simulink model "comprehensive_model_with_rocks_trial"  (R2019a)
settings: Solver=FixedStepAuto  StartTime=0.0  StopTime=15  FixedStep=0.001  RelTol=1e-3
PreLoadFcn:
  | load('tumbleweed_constants.mat')
values from neighbouring files (symbols this model uses):
  Ar = 0.785398163397    [tumbleweed_constants.mat]
  CD = 0.8    [tumbleweed_constants.mat]
  d = 0.65    [tumbleweed_constants.mat]
  g = 9.81    [tumbleweed_constants.mat]
  Ixx = 1.29    [tumbleweed_constants.mat]
  Iyy = 1.29    [tumbleweed_constants.mat]
  Izz = 1.29    [tumbleweed_constants.mat]
  m = 1    [tumbleweed_constants.mat]
  maxr = 0.45    [tumbleweed_constants.mat]
  mf = 14    [tumbleweed_constants.mat]
  minr = 0.2    [tumbleweed_constants.mat]
  mu0 = 0.02    [tumbleweed_constants.mat]
  muk = 0.5    [tumbleweed_constants.mat]
  must = 0.8    [tumbleweed_constants.mat]
  R = cylR*ones(size(Theta,1),size(Theta,2))    [d3_animate.m]    (also in tumbleweed_constants.mat = 0.5)
  rest_coeff = 0.6    [tumbleweed_constants.mat]
  rho = 1.2    [tumbleweed_constants.mat]
  ts = 0.5    [tumbleweed_constants.mat]
  v_thres = 0.0001    [tumbleweed_constants.mat]
  vmax = 0.2    [tumbleweed_constants.mat]
  YY = 50    [tumbleweed_constants.mat]
libraries: simulink x2
(part 4 of 9)

== matlab function comprehensive_model_with_rocks_trial/bouncing_model/onsurface_model/MATLAB Function5 ==
  data: t input; jAp input; states_from_memory input; states_internal input; r_AO0 input; roll_reset_flag input; surf_num_memory input; surf_num_internal input; rock_cents input; rock_radi input; switch_t input; OwT_OvAO0 output; R parameter; r_AO0 output; q output; roll_reset_flag output; reset_states output; reset_states input; surf_num output
function  [OwT_OvAO0, r_AO0, q,roll_reset_flag,reset_states,surf_num] = init_cond_supp(t,jAp, states_from_memory, states_internal,r_AO0, roll_reset_flag,surf_num_memory,surf_num_internal,rock_cents,rock_radi,switch_t, R, reset_states)
if t == 115.737
    disp(t)
end
if (t - switch_t) == 0
    roll_reset_flag = 1;
    states0 = states_from_memory;
    surf_num = surf_num_memory;
else
    states0 = states_internal;
    if mod(t,0.001) == 0
        surf_num = surf_num_internal;
    else
        surf_num = surf_num_memory;
    end
end
    
O_w_T = states0(1:3,1);
O_v_TO = states0(4:6,1);
r_TO = states0(7:9,1);
q = states0(10:13,1);
rock_radi = rock_radi.';


kO = [0;0;1];
jO = [0;1;0];
iO = [1;0;0];
point_on_surf =  zeros(2,1);
smallest_dist = 0;
if (roll_reset_flag == 1 && surf_num == 0)
    [point_on_surf, smallest_dist] = dist_calc(r_TO);
%     point_on_surf = [r_TO(1);r_TO(2)];
%     smallest_dist = r_TO(3);
    z_c = surf_eq(point_on_surf(1),point_on_surf(2),r_TO);
    r_AO0 = [point_on_surf;z_c];
elseif (roll_reset_flag == 1 && surf_num > 0)
    kR = (r_TO - rock_cents(:,surf_num))/norm(r_TO -  rock_cents(:,surf_num));
    point_on_rock = rock_cents(:,surf_num) + rock_radi(1,surf_num)*kR;
    r_AO0 = point_on_rock;
end

if surf_num == 0
    par_diffs = par_diffs_calc(r_AO0);
else
    par_diffs = rock_pardiffs_calc(r_AO0, rock_cents(:,surf_num)');
end

vx = O_v_TO(1); vy = O_v_TO(2); vz = O_v_TO(3);
fx = par_diffs(1);
fy = par_diffs(2);
fz = par_diffs(3);
fxx = par_diffs(4);
fxy = par_diffs(5);
fxz = par_diffs(6);
fyy = par_diffs(7);
fyz = par_diffs(8);
fzz = par_diffs(9);
fxxx = par_diffs(10);
fxxy = par_diffs(11);
fxxz = par_diffs(12);
fxyy = par_diffs(13);
fxyz = par_diffs(14);
fxzz = par_diffs(15);
fyyy = par_diffs(16);
fyyz = par_diffs(17);
fyzz = par_diffs(18);
fzzz = par_diffs(19);




q0 = q(1); q1 = q(2); q2 = q(3); q3 = q(4);


T_c_O = [q0^2 + q1^2 - q2^2 - q3^2, 2*(q1*q2 + q0*q3), 2*(q1*q3 - q0*q2);...
       2*(q1*q2 - q0*q3), q0^2 - q1^2 + q2^2 - q3^2, 2*(q2*q3 + q0*q1);...
       2*(q1*q3 + q0*q2), 2*(q2*q3 - q0*q1), q0^2 - q1^2 - q2^2 + q3^2];

c11 = T_c_O(1,1);c12 = T_c_O(1,2); c13 = T_c_O(1,3);
c21 = T_c_O(2,1);c22 = T_c_O(2,2); c23 = T_c_O(2,3);
c31 = T_c_O(3,1);c32 = T_c_O(3,2); c33 = T_c_O(3,3);




%z - cos(x/4)-1 = 0;
%- x^2 - y^2 = 0;

if(abs(fx)<=1e-20 && abs(fy) <= 1e-20)
    kA = kO;
    O_c_A = eye(3);
    A_c_O = eye(3);
    flag = 1;
else
    kA = [fx;fy;fz]/norm([fx;fy;fz]);
    jA = cross(kO,kA)/norm(cross(kO,kA));
    flag = 1;
    if((jAp.')*(jA) < 0)
        jA = -jA;
        flag = 2;
    end
    iA = cross(jA,kA);
    A_c_O = [iA'*iO, iA'*jO, iA'*kO; jA'*iO, jA'*jO, jA'*kO; kA'*iO, kA'*jO, kA'*kO];
    O_c_A = transpose(A_c_O);
end


if flag == 1
    
% OvAO_coeffs = ...
% [fx, fy, fz;...
% ((fx*fz*(fx^2 + fy^2 + fz^2)^(3/2) - R*fxz*(fx^2 + fy^2)^2 + R*fx*fxx*fz^3 + R*fxy*fy*fz^3 - R*fxz*fz^2*(fx^2 + fy^2) + R*fx*fxx*fz*(fx^2 + fy^2) + R*fxy*fy*fz*(fx^2 + fy^2))/((fx^2 + fy^2)^(1/2)*(fx^2 + fy^2 + fz^2)^2)),            ((fy*fz*(fx^2 + fy^2 + fz^2)^(3/2) - R*fyz*(fx^2 + fy^2)^2 + R*fx*fxy*fz^3 + R*fy*fyy*fz^3 - R*fyz*fz^2*(fx^2 + fy^2) + R*fx*fxy*fz*(fx^2 + fy^2) + R*fy*fyy*fz*(fx^2 + fy^2))/((fx^2 + fy^2)^(1/2)*(fx^2 + fy^2 + fz^2)^2)),               ((R*fx*fxz*fz^3 - R*fzz*(fx^2 + fy^2)^2 - (fx^2 + fy^2)*(fx^2 + fy^2 + fz^2)^(3/2) + R*fy*fyz*fz^3 - R*fz^2*fzz*(fx^2 + fy^2) + R*fx*fxz*fz*(fx^2 + fy^2) + R*fy*fyz*fz*(fx^2 + fy^2))/((fx^2 + fy^2)^(1/2)*(fx^2 + fy^2 + fz^2)^2));...
% (-(fy*(fx^2 + fy^2 + fz^2)^(1/2) - R*fx*fxy + R*fxx*fy)/((fx^2 + fy^2)^(1/2)*(fx^2 + fy^2 + fz^2)^(1/2))),                                                                                                                               ((fx*(fx^2 + fy^2 + fz^2)^(1/2) + R*fx*fyy - R*fxy*fy)/((fx^2 + fy^2)^(1/2)*(fx^2 + fy^2 + fz^2)^(1/2))),                                                                                                                                   ((R*fx*fyz - R*fxz*fy)/((fx^2 + fy^2)^(1/2)*(fx^2 + fy^2 + fz^2)^(1/2)))];
% 
% OvAO_consts = ...
% [0;...
% - (fx*fz*vx*(fx^2 + fy^2 + fz^2)^(3/2) - vz*(fx^2 + fy^2)*(fx^2 + fy^2 + fz^2)^(3/2) + fy*fz*vy*(fx^2 + fy^2 + fz^2)^(3/2))/((fx^2 + fy^2)^(1/2)*(fx^2 + fy^2 + fz^2)^2);...
% - (fx*vy*(fx^2 + fy^2 + fz^2)^(1/2) - fy*vx*(fx^2 + fy^2 + fz^2)^(1/2))/((fx^2 + fy^2)^(1/2)*(fx^2 + fy^2 + fz^2)^(1/2))];
%   

OvAO_coeffs = ...
 [(((fx^2 + fy^2 + fz^2)^(3/2) + R*fxx*fy^2 + R*fxx*fz^2 - R*fx*fxy*fy - R*fx*fxz*fz)/(fx^2 + fy^2 + fz^2)^(3/2)),       ((R*fxy*fy^2 - R*fx*fyy*fy + R*fxy*fz^2 - R*fx*fyz*fz)/(fx^2 + fy^2 + fz^2)^(3/2)),                                     ((R*fxz*fy^2 - R*fx*fyz*fy + R*fxz*fz^2 - R*fx*fzz*fz)/(fx^2 + fy^2 + fz^2)^(3/2));...
 ((R*fxy*fx^2 - R*fxx*fy*fx + R*fxy*fz^2 - R*fxz*fy*fz)/(fx^2 + fy^2 + fz^2)^(3/2)),                                     (((fx^2 + fy^2 + fz^2)^(3/2) + R*fx^2*fyy + R*fyy*fz^2 - R*fx*fxy*fy - R*fy*fyz*fz)/(fx^2 + fy^2 + fz^2)^(3/2)),        ((R*fyz*fx^2 - R*fxz*fy*fx + R*fyz*fz^2 - R*fy*fzz*fz)/(fx^2 + fy^2 + fz^2)^(3/2));...
 ((R*fxz*fx^2 - R*fxx*fz*fx + R*fxz*fy^2 - R*fxy*fz*fy)/(fx^2 + fy^2 + fz^2)^(3/2)),                                     ((R*fyz*fx^2 - R*fxy*fz*fx + R*fyz*fy^2 - R*fyy*fz*fy)/(fx^2 + fy^2 + fz^2)^(3/2)),                                     (((fx^2 + fy^2 + fz^2)^(3/2) + R*fx^2*fzz + R*fy^2*fzz - R*fx*fxz*fz - R*fy*fyz*fz)/(fx^2 + fy^2 + fz^2)^(3/2))];

OvAO_consts = ...
  [-vx;...
   -vy;...
   -vz];


else
    
% OvAO_coeffs = ...  
% [fx, fy, fz;...
% (-(fx*fz*(fx^2 + fy^2 + fz^2)^(3/2) - R*fxz*(fx^2 + fy^2)^2 + R*fx*fxx*fz^3 + R*fxy*fy*fz^3 - R*fxz*fz^2*(fx^2 + fy^2) + R*fx*fxx*fz*(fx^2 + fy^2) + R*fxy*fy*fz*(fx^2 + fy^2))/((fx^2 + fy^2)^(1/2)*(fx^2 + fy^2 + fz^2)^2)),           (-(fy*fz*(fx^2 + fy^2 + fz^2)^(3/2) - R*fyz*(fx^2 + fy^2)^2 + R*fx*fxy*fz^3 + R*fy*fyy*fz^3 - R*fyz*fz^2*(fx^2 + fy^2) + R*fx*fxy*fz*(fx^2 + fy^2) + R*fy*fyy*fz*(fx^2 + fy^2))/((fx^2 + fy^2)^(1/2)*(fx^2 + fy^2 + fz^2)^2)),              (-(R*fx*fxz*fz^3 - R*fzz*(fx^2 + fy^2)^2 - (fx^2 + fy^2)*(fx^2 + fy^2 + fz^2)^(3/2) + R*fy*fyz*fz^3 - R*fz^2*fzz*(fx^2 + fy^2) + R*fx*fxz*fz*(fx^2 + fy^2) + R*fy*fyz*fz*(fx^2 + fy^2))/((fx^2 + fy^2)^(1/2)*(fx^2 + fy^2 + fz^2)^2));...
% ((fy*(fx^2 + fy^2 + fz^2)^(1/2) - R*fx*fxy + R*fxx*fy)/((fx^2 + fy^2)^(1/2)*(fx^2 + fy^2 + fz^2)^(1/2))),                                                                                                                                (-(fx*(fx^2 + fy^2 + fz^2)^(1/2) + R*fx*fyy - R*fxy*fy)/((fx^2 + fy^2)^(1/2)*(fx^2 + fy^2 + fz^2)^(1/2))),                                                                                                                                  (-(R*fx*fyz - R*fxz*fy)/((fx^2 + fy^2)^(1/2)*(fx^2 + fy^2 + fz^2)^(1/2)))];      
%  
% OvAO_consts = ...
% [0;...
% (fx*fz*vx*(fx^2 + fy^2 + fz^2)^(3/2) - vz*(fx^2 + fy^2)*(fx^2 + fy^2 + fz^2)^(3/2) + fy*fz*vy*(fx^2 + fy^2 + fz^2)^(3/2))/((fx^2 + fy^2)^(1/2)*(fx^2 + fy^2 + fz^2)^2);...
% (fx*vy*(fx^2 + fy^2 + fz^2)^(1/2) - fy*vx*(fx^2 + fy^2 + fz^2)^(1/2))/((fx^2 + fy^2)^(1/2)*(fx^2 + fy^2 + fz^2)^(1/2))];

OvAO_coeffs = ...
   [(((fx^2 + fy^2 + fz^2)^(3/2) + R*fxx*fy^2 + R*fxx*fz^2 - R*fx*fxy*fy - R*fx*fxz*fz)/(fx^2 + fy^2 + fz^2)^(3/2)),              ((R*fxy*fy^2 - R*fx*fyy*fy + R*fxy*fz^2 - R*fx*fyz*fz)/(fx^2 + fy^2 + fz^2)^(3/2)),                                     ((R*fxz*fy^2 - R*fx*fyz*fy + R*fxz*fz^2 - R*fx*fzz*fz)/(fx^2 + fy^2 + fz^2)^(3/2));...
    ((R*fxy*fx^2 - R*fxx*fy*fx + R*fxy*fz^2 - R*fxz*fy*fz)/(fx^2 + fy^2 + fz^2)^(3/2)),                                           (((fx^2 + fy^2 + fz^2)^(3/2) + R*fx^2*fyy + R*fyy*fz^2 - R*fx*fxy*fy - R*fy*fyz*fz)/(fx^2 + fy^2 + fz^2)^(3/2)),        ((R*fyz*fx^2 - R*fxz*fy*fx + R*fyz*fz^2 - R*fy*fzz*fz)/(fx^2 + fy^2 + fz^2)^(3/2));...
    ((R*fxz*fx^2 - R*fxx*fz*fx + R*fxz*fy^2 - R*fxy*fz*fy)/(fx^2 + fy^2 + fz^2)^(3/2)),                                           ((R*fyz*fx^2 - R*fxy*fz*fx + R*fyz*fy^2 - R*fyy*fz*fy)/(fx^2 + fy^2 + fz^2)^(3/2)),                                     (((fx^2 + fy^2 + fz^2)^(3/2) + R*fx^2*fzz + R*fy^2*fzz - R*fx*fxz*fz - R*fy*fyz*fz)/(fx^2 + fy^2 + fz^2)^(3/2))];

OvAO_consts = ...
  [-vx;...
   -vy;...
   -vz];

end

if (abs(fx) <= 1e-20 && abs(fy) <= 1e-20 )
    O_v_AO = O_v_TO;
else
O_v_AO = -inv(OvAO_coeffs)*OvAO_consts;
end
O_v_AOa = A_c_O*O_v_AO;
if O_v_AOa(3) <= 0.008 && O_v_AOa(3) >= -0.008
    O_v_AOa(3) = 0;
    O_v_AO = O_c_A*O_v_AOa;
end
% if norm([O_v_AO(1);O_v_AO(2)]) < 0.00 
%     O_v_AO(1) = 0;
%     O_v_AO(2) = 0;
% end
OwT_OvAO0 = [O_w_T;O_v_AO];
if roll_reset_flag == 1
 reset_states = [O_w_T;O_v_AO;r_AO0;q];
end

end




function rock_pardiffs = rock_pardiffs_calc(point_on_rock, rock_center)
r_RO = point_on_rock; x_c = r_RO(1); y_c = r_RO(2); z_c = r_RO(3);
r_CO = rock_center';
fx = 2*(x_c - r_CO(1));
fy = 2*(y_c - r_CO(2));
fz = 2*(z_c - r_CO(3));
fxx = 2;
fxy = 0;
fxz = 0;
fyy = 2;
fyz = 0;
fzz = 2;
fxxx = 0;
fxxy = 0;
fxxz = 0;
fxyy = 0;
fxyz = 0;
fxzz = 0;
fyyy = 0;
fyyz = 0;
fyzz = 0;
fzzz = 0;
rock_pardiffs = [fx;fy;fz;fxx;fxy;fxz;fyy;fyz;fzz;fxxx;fxxy;fxxz;fxyy;fxyz;fxzz;fyyy;fyyz;fyzz;fzzz];
end



function par_diffs = par_diffs_calc(r_AO)

x_c = r_AO(1);
y_c = r_AO(2);
z_c = r_AO(3);

fx = 0;%4*exp(- (x_c - 5)^2/36 - y_c^2/36)*(x_c/18 - 5/18) - 6*exp(- (x_c - 5)^2/16 - y_c^2/16)*(x_c/8 - 5/8);
fy = 0;%(2*y_c*exp(- (x_c - 5)^2/36 - y_c^2/36))/9 - (3*y_c*exp(- (x_c - 5)^2/16 - y_c^2/16))/4;
fz = 1;
fxx = 0;%(2*exp(- (x_c - 5)^2/36 - y_c^2/36))/9 - (3*exp(- (x_c - 5)^2/16 - y_c^2/16))/4 + 6*exp(- (x_c - 5)^2/16 - y_c^2/16)*(x_c/8 - 5/8)^2 - 4*exp(- (x_c - 5)^2/36 - y_c^2/36)*(x_c/18 - 5/18)^2;
fxy = 0;%(3*y_c*exp(- (x_c - 5)^2/16 - y_c^2/16)*(x_c/8 - 5/8))/4 - (2*y_c*exp(- (x_c - 5)^2/36 - y_c^2/36)*(x_c/18 - 5/18))/9;
fxz = 0;
fyy = 0;%(2*exp(- (x_c - 5)^2/36 - y_c^2/36))/9 - (3*exp(- (x_c - 5)^2/16 - y_c^2/16))/4 + (3*y_c^2*exp(- (x_c - 5)^2/16 - y_c^2/16))/32 - (y_c^2*exp(- (x_c - 5)^2/36 - y_c^2/36))/81;
fyz = 0;
fzz = 0;
fxxx = 0;%(3*exp(- (x_c - 5)^2/16 - y_c^2/16)*(x_c/8 - 5/8))/4 + 6*exp(- (x_c - 5)^2/16 - y_c^2/16)*(x_c/32 - 5/32) - (2*exp(- (x_c - 5)^2/36 - y_c^2/36)*(x_c/18 - 5/18))/9 - 4*exp(- (x_c - 5)^2/36 - y_c^2/36)*(x_c/162 - 5/162) - 6*exp(- (x_c - 5)^2/16 - y_c^2/16)*(x_c/8 - 5/8)^3 + 4*exp(- (x_c - 5)^2/36 - y_c^2/36)*(x_c/18 - 5/18)^3;
fxxy = 0;%(3*y_c*exp(- (x_c - 5)^2/16 - y_c^2/16))/32 - (y_c*exp(- (x_c - 5)^2/36 - y_c^2/36))/81 - (3*y_c*exp(- (x_c - 5)^2/16 - y_c^2/16)*(x_c/8 - 5/8)^2)/4 + (2*y_c*exp(- (x_c - 5)^2/36 - y_c^2/36)*(x_c/18 - 5/18)^2)/9;
fxxz = 0;
fxyy = 0;%(3*exp(- (x_c - 5)^2/16 - y_c^2/16)*(x_c/8 - 5/8))/4 - (2*exp(- (x_c - 5)^2/36 - y_c^2/36)*(x_c/18 - 5/18))/9 - (3*y_c^2*exp(- (x_c - 5)^2/16 - y_c^2/16)*(x_c/8 - 5/8))/32 + (y_c^2*exp(- (x_c - 5)^2/36 - y_c^2/36)*(x_c/18 - 5/18))/81;
fxyz = 0;
fxzz = 0;
fyyy = 0;%(9*y_c*exp(- (x_c - 5)^2/16 - y_c^2/16))/32 - (y_c*exp(- (x_c - 5)^2/36 - y_c^2/36))/27 - (3*y_c^3*exp(- (x_c - 5)^2/16 - y_c^2/16))/256 + (y_c^3*exp(- (x_c - 5)^2/36 - y_c^2/36))/1458;
fyyz = 0;
fyzz = 0;
fzzz = 0;

% fx = -x_c;
% fy = 1;
% fz = z_c;
% fxx = -1;
% fxy = 0;
% fxz = 0;
% fyy = 0;
% fyz = 0;
% fzz = 1;
% fxxx = 0;
% fxxy = 0;
% fxxz = 0;
% fxyy = 0;
% fxyz = 0;
% fxzz = 0;
% fyyy = 0;
% fyyz = 0;
% fyzz = 0;
% fzzz = 0;

par_diffs = [fx;fy;fz;fxx;fxy;fxz;fyy;fyz;fzz;fxxx;fxxy;fxxz;fxyy;fxyz;fxzz;fyyy;fyyz;fyzz;fzzz];
end

function z_c = surf_eq(x_c, y_c, r_TO)
% if r_TO(3) >= 0
%     if x_c^2 - 2*y_c < 0
%         z_c = 0;
%     else
%     z_c = sqrt(x_c^2 - 2*y_c);
%     end
% else
%     if x_c^2 - 2*y_c < 0
%         z_c = 0;
%     else
%     z_c = -sqrt(x_c^2 - 2*y_c);
%     end
% end
z_c = 0;%(4*exp(-((x_c-5)^2 + (y_c)^2)/(6^2))-6*exp(-((x_c-5)^2 + (y_c)^2)/(4^2)));%(-1*exp(-((x_c - 10)^2 + (y_c - 10)^2)/2^2) -5*exp(-((x_c - 10)^2 + (y_c - 15)^2)/5^2) + 5*exp(-((x_c - 10)^2 + (y_c + 10)^2)/5^2) - 3*exp(-((x_c - 20)^2 + (y_c +5)^2)/4^2) - 5*exp(-((x_c - 40)^2 + (y_c -10)^2)/6^2));
end

== matlab function comprehensive_model_with_rocks_trial/bouncing_model/onsurface_model/MATLAB Function6 ==
  data: t input; switch_t input; states0 output; states input; states_from_memory input; point_on_rock output; rock_cents input; rock_radi input; rock_pardiffs output; rock_coll_flag output; R parameter; jAp input; surf_num input; surf_num output; roll_reset_flag input; reset_states input
function [states0, point_on_rock, rock_pardiffs, rock_coll_flag, surf_num] = collision_check(t, switch_t, states, states_from_memory,rock_cents, rock_radi,R, jAp, surf_num,roll_reset_flag,reset_states)
if t >= 88.46
    disp(t)
end
if (t - switch_t) == 0
    states0 = states_from_memory;
    O_w_T = states0(1:3,1);
    O_v_TO = states0(4:6,1);
    q = states0(10:13,1);
    r_TO = states0(7:9,1);
else
  states0 = states;
    if roll_reset_flag == 1
        states0 = reset_states;
    end
    O_w_T = states0(1:3,1);
    O_v_AO = states0(4:6,1);
    q = states0(10:13,1);
    r_AO = states0(7:9,1);
    [r_TO,  O_v_TO] = calc_OvTO_rTO(r_AO, O_v_AO, surf_num,rock_cents, jAp, R);
 end



rock_radi = rock_radi';
rock_coll_flag = 0;
rock_ind = 0;
kO = [0;0;1];
jO = [0;1;0];
iO = [1;0;0];

for i = 1:size(rock_cents,2)
    if i ~= surf_num
    if norm(r_TO - rock_cents(:,i)) <= rock_radi(1,i) + R + 0.001
        kR = (r_TO - rock_cents(:,i))/norm(r_TO -  rock_cents(:,i));   
       if(abs(kR(1))<=1e-10 && abs(kR(2))<=1e-10)
            kR = kO;
            jR = jO;
            iR = iO;
            O_c_R = eye(3);
            R_c_O = eye(3);
            flag = 1;
       else
        jR = cross(kO,kR)/norm(cross(kO,kR));
        flag = 1;
        if((jAp.')*(jR) < 0)
            jR = -jR;
            flag = 2;
        end
        iR = cross(jR,kR);
        R_c_O = [iR'*iO, iR'*jO, iR'*kO; jR'*iO, jR'*jO, jR'*kO; kR'*iO, kR'*jO, kR'*kO];
        O_c_R = transpose(R_c_O);
        end
    O_v_TOr = R_c_O*O_v_TO;  
        if O_v_TOr(3)< -0.001
                rock_coll_flag = 1;
                rock_ind = i;
        end
    end
    end
end

point_on_surf = [0;0];z_c = 0;
 smallest_dist = 0;
if surf_num ~= 0
     [point_on_surf, smallest_dist] = dist_calc(r_TO);
%     point_on_surf = [r_TO(1);r_TO(2)];
%     smallest_dist = r_TO(3);
    z_c = surf_eq(point_on_surf(1),point_on_surf(2),r_TO);
    if norm(r_TO - [point_on_surf;z_c]) <= R + 0.001  
                rock_coll_flag = 1;
                rock_ind = 0;
    end
end

if rock_coll_flag == 1
    if rock_ind == 0
        point_on_rock  = [point_on_surf;z_c];
        rock_pardiffs = surf_pardiffs_calc(point_on_rock);
%         fx = rock_pardiffs(1);
%         fy = rock_pardiffs(2);
%         fz = rock_pardiffs(3);
%         if(abs(fx)<=1e-20 && abs(fy) <= 1e-20)
%             kR = kO;
%             jR = jO;
%             iR = iO;
%             O_c_R = eye(3);
%             R_c_O = eye(3);
%         else
%             kR = [fx;fy;fz]/norm([fx;fy;fz]);
%             jR = cross(kO,kR)/norm(cross(kO,kR));
%         if((jRp.')*(jR) < 0)
%             jR = -jR;
%         end
%         iR = cross(jR,kR);
%         R_c_O = [iR'*iO, iR'*jO, iR'*kO; jR'*iO, jR'*jO, jR'*kO; kR'*iO, kR'*jO, kR'*kO];
%         O_c_R = transpose(R_c_O);
%         end
%         O_v_TOr = R_c_O*O_v_TO;  
%         if abs(O_v_TOr(3))<=0.001 && mod(t,0.001) == 0
%             surf_num = 0;
%         end
    if mod(t,0.001) == 0
        surf_num = 0;
    end
    else
        kR = (r_TO - rock_cents(:,rock_ind))/norm(r_TO -  rock_cents(:,rock_ind));
        point_on_rock = rock_cents(:,rock_ind) + rock_radi(1,rock_ind)*kR;
        rock_pardiffs = rock_pardiffs_calc(point_on_rock, rock_cents(:,rock_ind));
    end
else
    point_on_rock = [0;0;0];
    rock_pardiffs = zeros(19,1);
end


states0 = [O_w_T; O_v_TO; r_TO; q];
end









function [r_TO,  O_v_TO] = calc_OvTO_rTO(r_AO, O_v_AO, surf_num,rock_cents, jAp, R)
%change this everytime u change the function

x_dot = O_v_AO(1);
y_dot = O_v_AO(2);
z_dot = O_v_AO(3);

kO = [0;0;1];
jO = [0;1;0];
iO = [1;0;0];

%z - cos(x/4)-1 = 0;
%- x^2 - y^2 = 0;


if surf_num == 0
    par_diffs = surf_pardiffs_calc(r_AO);
else
    rock_center = rock_cents(:,surf_num);
    par_diffs = rock_pardiffs_calc(r_AO, rock_center);
end
fx = par_diffs(1);
fy = par_diffs(2);
fz = par_diffs(3);
fxx = par_diffs(4);
fxy = par_diffs(5);
fxz = par_diffs(6);
fyy = par_diffs(7);
fyz = par_diffs(8);
fzz = par_diffs(9);
fxxx = par_diffs(10);
fxxy = par_diffs(11);
fxxz = par_diffs(12);
fxyy = par_diffs(13);
fxyz = par_diffs(14);
fxzz = par_diffs(15);
fyyy = par_diffs(16);
fyyz = par_diffs(17);
fyzz = par_diffs(18);
fzzz = par_diffs(19);


if(abs(fx)<=1e-20 && abs(fy) <= 1e-20)
    kA = kO;
    jA = jO;
    O_c_A = eye(3);
    A_c_O = eye(3);
    flag = 1;
else
    kA = [fx;fy;fz]/norm([fx;fy;fz]);
    jA = cross(kO,kA)/norm(cross(kO,kA));
    flag = 1;
    if((jAp.')*(jA) < 0)
        jA = -jA;
        flag = 2;
    end
    iA = cross(jA,kA);
    A_c_O = [iA'*iO, iA'*jO, iA'*kO; jA'*iO, jA'*jO, jA'*kO; kA'*iO, kA'*jO, kA'*kO];
    O_c_A = transpose(A_c_O);
end
if flag == 1
    O_w_A = ...
    [-(fx*fxy*x_dot - fy*fxx*x_dot + fx*fyy*y_dot - fy*fxy*y_dot + fx*fyz*z_dot - fy*fxz*z_dot)/((fx^2 + fy^2)^(1/2)*(fx^2 + fy^2 + fz^2)^(1/2));...
     -(fx^2*fxz*x_dot + fy^2*fxz*x_dot + fx^2*fyz*y_dot + fy^2*fyz*y_dot + fx^2*fzz*z_dot + fy^2*fzz*z_dot - fx*fxx*fz*x_dot - fy*fz*fxy*x_dot - fx*fz*fxy*y_dot - fy*fz*fyy*y_dot - fx*fz*fxz*z_dot - fy*fz*fyz*z_dot)/((fx^2 + fy^2)^(1/2)*(fx^2 + fy^2 + fz^2));...
     (fz*(fx*fxy*x_dot - fy*fxx*x_dot + fx*fyy*y_dot - fy*fxy*y_dot + fx*fyz*z_dot - fy*fxz*z_dot))/((fx^2 + fy^2)*(fx^2 + fy^2 + fz^2)^(1/2))];
else
    O_w_A = ...
    [(fx*fxy*x_dot - fy*fxx*x_dot + fx*fyy*y_dot - fy*fxy*y_dot + fx*fyz*z_dot - fy*fxz*z_dot)/((fx^2 + fy^2)^(1/2)*(fx^2 + fy^2 + fz^2)^(1/2));...
     (fx^2*fxz*x_dot + fy^2*fxz*x_dot + fx^2*fyz*y_dot + fy^2*fyz*y_dot + fx^2*fzz*z_dot + fy^2*fzz*z_dot - fx*fxx*fz*x_dot - fy*fz*fxy*x_dot - fx*fz*fxy*y_dot - fy*fz*fyy*y_dot - fx*fz*fxz*z_dot - fy*fz*fyz*z_dot)/((fx^2 + fy^2)^(1/2)*(fx^2 + fy^2 + fz^2));...
     (fz*(fx*fxy*x_dot - fy*fxx*x_dot + fx*fyy*y_dot - fy*fxy*y_dot + fx*fyz*z_dot - fy*fxz*z_dot))/((fx^2 + fy^2)*(fx^2 + fy^2 + fz^2)^(1/2))];
end
if (abs(fx) <= 1e-20 && abs(fy) <= 1e-20)
    O_w_A = [0;0;0];
end
r_TO = r_AO + R*kA;

r_TA = [0;0;R];
O_v_TO = O_v_AO + O_c_A*cross(O_w_A, r_TA);
end










function rock_pardiffs = rock_pardiffs_calc(point_on_rock, rock_center)
r_RO = point_on_rock; x_c = r_RO(1); y_c = r_RO(2); z_c = r_RO(3);
r_CO = rock_center';
fx = 2*(x_c - r_CO(1));
fy = 2*(y_c - r_CO(2));
fz = 2*(z_c - r_CO(3));
fxx = 2;
fxy = 0;
fxz = 0;
fyy = 2;
fyz = 0;
fzz = 2;
fxxx = 0;
fxxy = 0;
fxxz = 0;
fxyy = 0;
fxyz = 0;
fxzz = 0;
fyyy = 0;
fyyz = 0;
fyzz = 0;
fzzz = 0;
rock_pardiffs = [fx;fy;fz;fxx;fxy;fxz;fyy;fyz;fzz;fxxx;fxxy;fxxz;fxyy;fxyz;fxzz;fyyy;fyyz;fyzz;fzzz];
end











function par_diffs = surf_pardiffs_calc(r_AO)
x_c = r_AO(1);
y_c = r_AO(2);
z_c = r_AO(3);

fx = 0;%4*exp(- (x_c - 5)^2/36 - y_c^2/36)*(x_c/18 - 5/18) - 6*exp(- (x_c - 5)^2/16 - y_c^2/16)*(x_c/8 - 5/8);
fy = 0;%(2*y_c*exp(- (x_c - 5)^2/36 - y_c^2/36))/9 - (3*y_c*exp(- (x_c - 5)^2/16 - y_c^2/16))/4;
fz = 1;
fxx = 0;%(2*exp(- (x_c - 5)^2/36 - y_c^2/36))/9 - (3*exp(- (x_c - 5)^2/16 - y_c^2/16))/4 + 6*exp(- (x_c - 5)^2/16 - y_c^2/16)*(x_c/8 - 5/8)^2 - 4*exp(- (x_c - 5)^2/36 - y_c^2/36)*(x_c/18 - 5/18)^2;
fxy = 0;%(3*y_c*exp(- (x_c - 5)^2/16 - y_c^2/16)*(x_c/8 - 5/8))/4 - (2*y_c*exp(- (x_c - 5)^2/36 - y_c^2/36)*(x_c/18 - 5/18))/9;
fxz = 0;
fyy = 0;%(2*exp(- (x_c - 5)^2/36 - y_c^2/36))/9 - (3*exp(- (x_c - 5)^2/16 - y_c^2/16))/4 + (3*y_c^2*exp(- (x_c - 5)^2/16 - y_c^2/16))/32 - (y_c^2*exp(- (x_c - 5)^2/36 - y_c^2/36))/81;
fyz = 0;
fzz = 0;
fxxx = 0;%(3*exp(- (x_c - 5)^2/16 - y_c^2/16)*(x_c/8 - 5/8))/4 + 6*exp(- (x_c - 5)^2/16 - y_c^2/16)*(x_c/32 - 5/32) - (2*exp(- (x_c - 5)^2/36 - y_c^2/36)*(x_c/18 - 5/18))/9 - 4*exp(- (x_c - 5)^2/36 - y_c^2/36)*(x_c/162 - 5/162) - 6*exp(- (x_c - 5)^2/16 - y_c^2/16)*(x_c/8 - 5/8)^3 + 4*exp(- (x_c - 5)^2/36 - y_c^2/36)*(x_c/18 - 5/18)^3;
fxxy = 0;%(3*y_c*exp(- (x_c - 5)^2/16 - y_c^2/16))/32 - (y_c*exp(- (x_c - 5)^2/36 - y_c^2/36))/81 - (3*y_c*exp(- (x_c - 5)^2/16 - y_c^2/16)*(x_c/8 - 5/8)^2)/4 + (2*y_c*exp(- (x_c - 5)^2/36 - y_c^2/36)*(x_c/18 - 5/18)^2)/9;
fxxz = 0;
fxyy = 0;%(3*exp(- (x_c - 5)^2/16 - y_c^2/16)*(x_c/8 - 5/8))/4 - (2*exp(- (x_c - 5)^2/36 - y_c^2/36)*(x_c/18 - 5/18))/9 - (3*y_c^2*exp(- (x_c - 5)^2/16 - y_c^2/16)*(x_c/8 - 5/8))/32 + (y_c^2*exp(- (x_c - 5)^2/36 - y_c^2/36)*(x_c/18 - 5/18))/81;
fxyz = 0;
fxzz = 0;
fyyy = 0;%(9*y_c*exp(- (x_c - 5)^2/16 - y_c^2/16))/32 - (y_c*exp(- (x_c - 5)^2/36 - y_c^2/36))/27 - (3*y_c^3*exp(- (x_c - 5)^2/16 - y_c^2/16))/256 + (y_c^3*exp(- (x_c - 5)^2/36 - y_c^2/36))/1458;
fyyz = 0;
fyzz = 0;
fzzz = 0;

par_diffs = [fx;fy;fz;fxx;fxy;fxz;fyy;fyz;fzz;fxxx;fxxy;fxxz;fxyy;fxyz;fxzz;fyyy;fyyz;fyzz;fzzz];
end







function z_c = surf_eq(x_c, y_c, r_TO)
% if r_TO(3) >= 0
%     if x_c^2 - 2*y_c < 0
%         z_c = 0;
%     else
%     z_c = sqrt(x_c^2 - 2*y_c);
%     end
% else
%     if x_c^2 - 2*y_c < 0
%         z_c = 0;
%     else
%     z_c = -sqrt(x_c^2 - 2*y_c);
%     end
% end
z_c = 0;%(4*exp(-((x_c-5)^2 + (y_c)^2)/(6^2))-6*exp(-((x_c-5)^2 + (y_c)^2)/(4^2)));%(-1*exp(-((x_c - 10)^2 + (y_c - 10)^2)/2^2) -5*exp(-((x_c - 10)^2 + (y_c - 15)^2)/5^2) + 5*exp(-((x_c - 10)^2 + (y_c + 10)^2)/5^2) - 3*exp(-((x_c - 20)^2 + (y_c +5)^2)/4^2) - 5*exp(-((x_c - 40)^2 + (y_c -10)^2)/6^2));
end

== matlab function comprehensive_model_with_rocks_trial/bouncing_model/onsurface_model/MATLAB Function7 ==
  data: angacc_linacc input; states input; u input; angacc_linacc output; O_c_A input; O_w_A input; O_v_AO input; FW input; par_diffs input; OalA_coeffs input; OalA_consts input; slip_flag input; FN input; R parameter; Ixx parameter; Iyy parameter; Izz parameter; m parameter; mf parameter; muk parameter; mu0 parameter; v_thres parameter; g parameter; FN output
function [angacc_linacc, FN] = slip_anglinacc_calc(angacc_linacc, states, u, O_c_A, O_w_A, O_v_AO, FW, par_diffs, OalA_coeffs, OalA_consts, slip_flag, FN,  R, Ixx, Iyy, Izz, m, mf, muk, mu0, v_thres, g)

if slip_flag == true
I_T = [Ixx,0,0;0,Iyy,0;0,0,Izz]; 
r_m1T = [u(1);0;0]; T_v_m1T = [u(7);0;0]; T_a_m1T = [u(13);0;0];
r_m2T = [u(2);0;0]; T_v_m2T = [u(8);0;0]; T_a_m2T = [u(14);0;0];
r_m3T = [0;u(3);0]; T_v_m3T = [0;u(9);0]; T_a_m3T = [0;u(15);0];
r_m4T = [0;u(4);0]; T_v_m4T = [0;u(10);0]; T_a_m4T = [0;u(16);0];
r_m5T = [0;0;u(5)]; T_v_m5T = [0;0;u(11)]; T_a_m5T = [0;0;u(17)];
r_m6T = [0;0;u(6)]; T_v_m6T = [0;0;u(12)]; T_a_m6T = [0;0;u(18)];
r_CMT = m*(r_m1T + r_m2T + r_m3T + r_m4T + r_m5T + r_m6T)/(6*m+mf);
T_v_CMT = m*(T_v_m1T + T_v_m2T + T_v_m3T + T_v_m4T + T_v_m5T + T_v_m6T)/(6*m+mf);
T_a_CMT = m*(T_a_m1T + T_a_m2T + T_a_m3T + T_a_m4T + T_a_m5T + T_a_m6T)/(6*m+mf);
r_CMTx = Vx(r_CMT);r_m1Tx = Vx(r_m1T);r_m2Tx = Vx(r_m2T);r_m3Tx = Vx(r_m3T);
r_m4Tx = Vx(r_m4T);r_m5Tx = Vx(r_m5T);r_m6Tx = Vx(r_m6T);

q0 = states(10); q1 = states(11); q2 = states(12); q3 = states(13);
T_c_O = [q0^2 + q1^2 - q2^2 - q3^2, 2*(q1*q2 + q0*q3), 2*(q1*q3 - q0*q2);...
       2*(q1*q2 - q0*q3), q0^2 - q1^2 + q2^2 - q3^2, 2*(q2*q3 + q0*q1);...
       2*(q1*q3 + q0*q2), 2*(q2*q3 - q0*q1), q0^2 - q1^2 - q2^2 + q3^2];
O_c_T = T_c_O.';
T_c_A = T_c_O*O_c_A;
A_c_O = transpose(O_c_A);
A_c_T = T_c_A';

r_TA = [0;0;R];
r_TAx = Vx(r_TA);
r_AT = [0;0;-R];
r_ATx = Vx(r_AT);

O_v_TO = [states(4);states(5);states(6)];
O_w_T = [states(1);states(2);states(3)];
O_w_Tx = Vx(O_w_T);
O_v_PO = O_v_TO + cross(O_c_T*O_w_T, O_c_A*r_AT);
O_w_Ax = Vx(O_w_A);



fx = par_diffs(1);
fy = par_diffs(2);
fz = par_diffs(3);
fxx = par_diffs(4);
fxy = par_diffs(5);
fxz = par_diffs(6);
fyy = par_diffs(7);
fyz = par_diffs(8);
fzz = par_diffs(9);
fxxx = par_diffs(10);
fxxy = par_diffs(11);
fxxz = par_diffs(12);
fxyy = par_diffs(13);
fxyz = par_diffs(14);
fxzz = par_diffs(15);
fyyy = par_diffs(16);
fyyz = par_diffs(17);
fyzz = par_diffs(18);
fzzz = par_diffs(19);

x_dot = O_v_AO(1); y_dot = O_v_AO(2); z_dot = O_v_AO(3);

O_vel_TO = A_c_O*O_v_AO + cross(O_w_A, r_TA);
u_TO = O_vel_TO(1);
v_TO = O_vel_TO(2);
w_TO = O_vel_TO(3);
murr = mu0*tanh(sqrt(u_TO^2 + v_TO^2 + w_TO^2)/v_thres); 
roll_rest_coeff = [1,0,-murr*u_TO/sqrt(u_TO^2 + v_TO^2);0,1,-murr*v_TO/sqrt(u_TO^2 + v_TO^2);0,0,1];
FG = [0;0;-(mf+6*m)*g];
FGA = A_c_O*FG;
FR  = -murr*norm(FGA'*[0;0;1])*[u_TO; v_TO; w_TO]/sqrt(u_TO^2 + v_TO^2 + w_TO^2);

eps = 0.025;
N = norm(FGA'*[0;0;1]);
f = 0.5;%0.5;
OwTz = (A_c_T*O_w_T)'*[0;0;1];
if(abs(OwTz) <= 1e-4)
    MzT = [0;0;0];
else
MzT = [0;0;-3*pi*N*f*eps*OwTz/(16*norm(OwTz))];%-mu*N*[0;0;1];
end

C11 = I_T - m*r_m1Tx*r_m1Tx - m*r_m2Tx*r_m2Tx - m*r_m3Tx*r_m3Tx - m*r_m4Tx*r_m4Tx - m*r_m5Tx*r_m5Tx - m*r_m6Tx*r_m6Tx;
C12 = (mf + 6*m)*r_CMTx*(T_c_O - T_c_A*r_TAx*OalA_coeffs);
C13 = - T_c_A*r_ATx*[-muk*((A_c_O*O_v_PO).'*([1;0;0]))/(norm(O_v_PO));-muk*((A_c_O*O_v_PO).'*([0;1;0]))/(norm(O_v_PO));1];
C21 = -(mf + 6*m)*r_CMTx;
C22 =  (mf + 6*m)*(T_c_O - T_c_A*r_TAx*OalA_coeffs);
C23 = -T_c_A*[-muk*((A_c_O*O_v_PO).'*([1;0;0]))/(norm(O_v_PO));-muk*((A_c_O*O_v_PO).'*([0;1;0]))/(norm(O_v_PO));1];
C31 = [0, 0, 0];
C32 = [fx, fy, fz];
C33 = 0;

if norm(O_v_PO) < 1e-3
    C13 = - T_c_A*r_ATx*[-muk*((A_c_O*O_v_TO).'*([1;0;0]))/(norm(O_v_TO));-muk*((A_c_O*O_v_TO).'*([0;1;0]))/(norm(O_v_TO));1];
    C23 = -T_c_A*[-muk*((A_c_O*O_v_TO).'*([1;0;0]))/(norm(O_v_TO));-muk*((A_c_O*O_v_TO).'*([0;1;0]))/(norm(O_v_TO));1];
end

D1 = r_CMTx*T_c_O*FG + T_c_A*MzT - O_w_Tx*I_T*O_w_T - m*cross(r_m1T,2*O_w_Tx*T_v_m1T + O_w_Tx*O_w_Tx*r_m1T)...
       - m*r_m2Tx*(T_a_m2T + 2*O_w_Tx*T_v_m2T + O_w_Tx*O_w_Tx*r_m2T)...
       - m*r_m3Tx*(T_a_m3T + 2*O_w_Tx*T_v_m3T + O_w_Tx*O_w_Tx*r_m3T)...
       - m*r_m4Tx*(T_a_m4T + 2*O_w_Tx*T_v_m4T + O_w_Tx*O_w_Tx*r_m4T)...
       - m*r_m5Tx*(T_a_m5T + 2*O_w_Tx*T_v_m5T + O_w_Tx*O_w_Tx*r_m5T)...
       - m*r_m6Tx*(T_a_m6T + 2*O_w_Tx*T_v_m6T + O_w_Tx*O_w_Tx*r_m6T)...
       + (mf + 6*m)*r_CMTx*T_c_A*r_TAx*OalA_consts - (mf + 6*m)*r_CMTx*T_c_A*O_w_Ax*O_w_Ax*r_TA;
D2 = T_c_O*FG + T_c_A*FR + T_c_O*FW -(mf + 6*m)*(T_a_CMT + 2*O_w_Tx*T_v_CMT + O_w_Tx*O_w_Tx*r_CMT) ...
    + (mf + 6*m)*T_c_A*r_TAx*OalA_consts - (mf + 6*m)*T_c_A*O_w_Ax*O_w_Ax*r_TA;
D3 = -(x_dot*(fxx*x_dot + fxy*y_dot + fxz*z_dot) + y_dot*(fxy*x_dot + fyy*y_dot + fyz*z_dot) + z_dot*(fxz*x_dot + fyz*y_dot + fzz*z_dot));
C = [C11,C12,C13;C21,C22,C23;C31,C32,C33]; D = [D1;D2;D3];
OalT_OaAO_FN = inv(C)*D;
O_al_T = OalT_OaAO_FN(1:3,1);
O_a_AO = OalT_OaAO_FN(4:6,1);
FN = OalT_OaAO_FN(7,1);

angacc_linacc = [O_al_T;O_a_AO];
end
end

== matlab function comprehensive_model_with_rocks_trial/bouncing_model/onsurface_model/MATLAB Function8 ==
  data: O_v_AO input; O_v_TO output; O_c_A input; O_w_A input; R parameter
function O_v_TO = OvTO_calc(O_v_AO, O_c_A, O_w_A, R)

r_TA = [0;0;R];
O_v_TO = O_v_AO + O_c_A*cross(O_w_A, r_TA);


end

== matlab function comprehensive_model_with_rocks_trial/bouncing_model/onsurface_model/MATLAB Function9 ==
  data: t input; states0 output size=13; roll_reset_flag output size=1; states input; u input; r_RO input; rock_coll_flag input; rock_pardiffs input; jRp input size=3; jR output size=3; rest_coeff parameter; m parameter; mf parameter; Ixx parameter; d parameter; R parameter; must parameter; muk parameter; Iyy parameter; Izz parameter
function [states0, roll_reset_flag, jR] = rock_collision_state_set(t,states,u, r_RO, rock_coll_flag, rock_pardiffs, jRp, rest_coeff, m, mf, Ixx, d, R, must, muk, Iyy, Izz)
%u1 u2 u3 u4 u5 u6 S1 S2 S3
roll_reset_flag = 0;
O_w_T = [states(1);states(2);states(3)];
O_v_TO = [states(4);states(5);states(6)];
r_TO = [states(7);states(8);states(9)];
q = [states(10);states(11);states(12);states(13)];
q0 = q(1); q1 = q(2); q2 = q(3); q3 = q(4);

        fx = rock_pardiffs(1,1); 
        fy = rock_pardiffs(2,1);
        fz = rock_pardiffs(3,1);
        kO = [0;0;1];
        iO = [1;0;0];
        jO = [0;1;0];

        if(abs(fx)<=1e-20 && abs(fy) <= 1e-20)
            kR = kO;
            jR = jO;
            iR = iO;
            O_c_R = eye(3);
            R_c_O = eye(3);
            flag = 1;
        else
        kR = [fx;fy;fz]/norm([fx;fy;fz]);
        jR = cross(kO,kR)/norm(cross(kO,kR));
        flag = 1;
        if((jRp.')*(jR) < 0)
            jR = -jR;
            flag = 2;
        end
        iR = cross(jR,kR);
        R_c_O = [iR'*iO, iR'*jO, iR'*kO; jR'*iO, jR'*jO, jR'*kO; kR'*iO, kR'*jO, kR'*kO];
        O_c_R = transpose(R_c_O);
        end
O_v_TOr = R_c_O*O_v_TO;       

if rock_coll_flag == 0
    jR = [0;1;0];
end
        
if mod(t,0.001) == 0 && rock_coll_flag == 1
 %%collision response
     
        T_c_O = [q0^2 + q1^2 - q2^2 - q3^2, 2*(q1*q2 + q0*q3), 2*(q1*q3 - q0*q2);...
        2*(q1*q2 - q0*q3), q0^2 - q1^2 + q2^2 - q3^2, 2*(q2*q3 + q0*q1);...
        2*(q1*q3 + q0*q2), 2*(q2*q3 - q0*q1), q0^2 - q1^2 - q2^2 + q3^2];
        O_c_T = T_c_O.';
       
        
        
        T_c_R = T_c_O*O_c_R;
        R_c_T = T_c_R.';
        
        l1 = u(1); l2 = u(2); l3 = u(3); l4 = u(4); l5 = u(5); l6 = u(6);
        L33 = Ixx + m*(l3^2 + l4^2 + l5^2 + l6^2);
        L11 = Iyy + m*(l1^2 + l2^2 + l5^2 + l6^2);
        L22 = Izz + m*(l3^2 + l4^2 + l1^2 + l2^2);
        L = R_c_T*[L33,0,0;0,L11,0;0,0,L22]*T_c_R;
        L11 = L(2,2);
        L22 = L(3,3);
        L33 = L(1,1);
        mT = mf +6*m;

        w = R_c_T*(O_w_T);
        v = R_c_O*O_v_TO;

        u3 = w(1,1);
        u2 = w(3,1);
        u1 = w(2,1);

        u6 = v(1,1);
        u5 = v(3,1);
        u4 = v(2,1);


        u5_n = -rest_coeff*u5;  

        roll_reset_flag = 1;
        r_TO = r_RO + R*kR;
        
        u2_n = u2;
        u3_n = (L33*u3 - mT*R*u4)/(mT*R^2 + L33);
        u4_n = -R*u3_n;
        u1_n = (L11*u1 + mT*R*u6)/(mT*R^2 + L11);
        u6_n = R*u1_n;
        S1 = mT*(u4_n - u4);
        S2 = mT*(u5_n - u5);
        S3 = mT*(u6_n - u6);

        if ~(sqrt(S1^2 + S3^2) < must*norm(S2))
            alpha = u4 + R*u3;
            gamma = u6 - R*u1;
            k1 = 1/mT + R^2/L11;
            k3 = 1/mT + R^2/L33;
            
            if abs(alpha) > 0
                S1 = S1solve(S2, muk,alpha, gamma, k1, k3); 
                S3 = gamma*S1/(alpha + (k3 - k1)*S1);
                u1_n = u1 - R*S3/L11;
                u3_n = u3 + R*S1/L33;
                u4_n = u4 + S1/mT;
                u6_n = u6 + S3/mT;
            else 
                S3 = S1solve(S2, muk, gamma, alpha, k3, k1);
                S1 = alpha*S3/(gamma + (k1 - k3)*S3);
                u1_n = u1 - R*S3/L11;
                u3_n = u3 + R*S1/L33;
                u4_n = u4 + S1/mT;
                u6_n = u6 + S3/mT;
            end
            
        end

        O_w_T = T_c_R*[u3_n;u1_n;u2_n];
        O_v_TO = O_c_R*[u6_n; u4_n; u5_n];
end

states0 = [O_w_T;O_v_TO;r_TO;q];

end
